simulink model "ICE_Tractor_KRAKER_etrailer_v2_3"  (R2023a)
settings: Solver=VariableStepAuto  StartTime=0.0  StopTime=tmax  FixedStep=dt  RelTol=1e-3  EnableMultiTasking=on
PreLoadFcn:
  | init_vehicle
  | init_SIMULATION_runfile
StartFcn:
  | tic
StopFcn:
  | toc
  | sim_stop_function
  | ICE_Etrailer_Simscape_MBM_plotting
values from neighbouring files (symbols this model uses):
  Arms = [100 200 300 400 500 600]    [init_BURGERS.m]    (also in init_KRAKER.m)
  brake_input = [0   tmax ... (first row only)    [init_vehicle.m]    (also in run_Circle.m = [0  tmax; run_Coastdown.m = [0  2  tmax; run_DoubleLaneChangeDriver.m = [0   2  tmax; run_MaxAcc.m = [0  2  tmax)
  chassis_length = 13.82    [init_BURGERS.m]    (also in init_KRAKER.m = 10.36)
  Diesel_density = 850    [init_BURGERS.m]    (also in init_KRAKER.m)
  Eff = [336.0 370.2 399.2 423.6 444.0 461.0 475.2 487.2 496.2 502.6 506.2 506.9 504.2 500.0 492.4 482.3 469.2 ; 271.0 278.2 285.5 292.8 300.0 307.0 313.7 320.0 325.9 331.5 336.7 341.5 345.9 350.0 353.7 357.0 360.0 ; 223.2 222.7 222.2 221.9 222.0 222.7 224.2 226.7 230.0 234.2 239.3 245.3 252.2 260.0 268.7 278.2 288.7 ; 227.6 221.7 216.8 212.9 210.0 208.1 207.2 207.3 208.5 210.7 214.0 218.3 223.6 230.0 237 ...(+640 chars)    [init_BURGERS.m]    (also in init_KRAKER.m)
  energyCapacity = 116.89    [init_BURGERS.m]    (also in init_KRAKER.m)
  etrailer_ON = 1    [init_SIMULATION_runfile.m]
  front_overhang = 1.620    (= 1.62)    [init_BURGERS.m]    (also in init_KRAKER.m = 1.305)
  G_diff = 1    [init_BURGERS.m]    (also in init_KRAKER.m = 6)
  initialSOC = 0.95    [init_BURGERS.m]    (also in init_KRAKER.m = 0.65)
  InputSwitch = 2    [init_SIMULATION_runfile.m]
  inverter_thermal_res = 0.017    [init_BURGERS.m]    (also in init_KRAKER.m)
  L_0f = 3.8    [init_vehicle.m]
  LD = 1    [init_vehicle.m]
  mass = mass_trailer    (= 11000)    [init_BURGERS.m]    (also in init_KRAKER.m = 7350; run_Statics_MF_MAT.m = (Fz_front_axle1+Fz_rear_axle1+       Fz_trailer1_axle1+Fz_tr; run_Statics_MF_TNO.m = (Fz_front_axle1+Fz_rear_axle1+       Fz_trailer1_axle1+Fz_tr)
  massload = 23000    [init_SIMULATION_runfile.m]
  MaxTrqOut = 525    [init_BURGERS.m]    (also in init_KRAKER.m = 950)
  outside_temp = 25    [init_BURGERS.m]    (also in init_KRAKER.m)
  pose_t0 = [0 0 0 0]    [init_vehicle.m]    (also in run_Circle.m; run_Coastdown.m; run_DoubleLaneChangeDriver.m; run_MaxAcc.m)
  Power_dissipation = [261 384 513 642; 552 783 1020 1260; 894 1233 1584 1956; 1300 1750 2200 2740; 1740 2300 2900 3550; 2250 2900 3650 4500]    [init_BURGERS.m]    (also in init_KRAKER.m)
  RPM = [400 500 600 700 800 900 1000 1100 1200 1300 1400 1500 1600 1700 1800 1900 2000]    [init_BURGERS.m]    (also in init_KRAKER.m)
  sp_t = 0.01    [init_vehicle.m]
  Std_Regen_Trq = 300    [init_BURGERS.m]    (also in init_KRAKER.m)
  steer_input = [0  tmax ... (first row only)    [init_vehicle.m]    (also in run_Circle.m = [0  2   10     13       tmax; run_Coastdown.m = [0 tmax; run_DoubleLaneChangeDriver.m = [0 tmax; run_MaxAcc.m = [0 tmax)
  steer_ratio = 20    [init_vehicle.m]
  steer_sens = 1    [init_vehicle.m]
  throttle_input = [0         tmax ... (first row only)    [init_vehicle.m]    (also in run_Circle.m; run_Coastdown.m = [0        10         10.0001 tmax; run_DoubleLaneChangeDriver.m = [0        tmax; run_MaxAcc.m = [0        tmax)
  tire_param_drive = simscape.multibody.tirread('DRIVE_315_70R22.5_9b_MF62.tir')    [init_vehicle.m]
  tire_param_steer = simscape.multibody.tirread('STEER_315_70R22.5_9b_MF62.tir')    [init_vehicle.m]
  tire_param_trailer = simscape.multibody.tirread('TRAILER_385_65R22.5_9b0_MF62.tir')    [init_vehicle.m]
  tire_width = 0.318    [init_vehicle.m]
  Torq = [0 250 500 750 1000 1250 1500 1750 1850 2000]    [init_BURGERS.m]    (also in init_KRAKER.m)
  trailer_ID = 1    [init_SIMULATION_runfile.m]
  v_0 = 1    [init_vehicle.m]
  Vdc = [200 400 600 800]    [init_BURGERS.m]    (also in init_KRAKER.m)
  Voc = 675    [init_BURGERS.m]    (also in init_KRAKER.m)
  Vx = 0    [init_vehicle.m]    (also in run_Circle.m = Vx_kmh/3.6; run_Coastdown.m = Vx_kmh/3.6; run_DoubleLaneChangeDriver.m = Vx_kmh/3.6; run_MaxAcc.m)
  Vx_input = [0  tmax ... (first row only)    [init_vehicle.m]    (also in run_Circle.m; run_Coastdown.m = [0 tmax; run_DoubleLaneChangeDriver.m = [0 tmax; run_MaxAcc.m = [0 tmax)
  wheelbase = 8.115    [init_BURGERS.m]    (also in init_KRAKER.m = 5.584)
undefined symbols (not defined in the file or in its folder): end_val, final_x, final_y, Floor, steer_path, X, Y, Z
libraries: sm_lib x367, nesl_utility x281, fl_lib x15, sdl_lib x2, robotalgslib x1, simulink_extras x1, batteryecm_lib x1, ee_lib x1, BatteryEstimators x1, CommercialVehicleLibrary2G x1
(part 10 of 14)

== system ICE_Tractor_KRAKER_etrailer_v2_3/Tractor_semitrailer /KRAKER e-trailer/Trailer axle 1/Wheel FR ==
  Bus Creator : BusCreator  Inputs=6
  Bus Creator2 : BusCreator  Inputs=3
  Demux : Demux  Outputs=3
  Demux1 : Demux  Outputs=3
  Geometry Transform : sm_lib/Frames and Transforms/Rigid Transform  TranslationMethod=None  TranslationStandardOffset=0  TranslationStandardOffsetUnits=m  TranslationStandardAxis=+Y  TranslationCartesianOffset=[0 0 0]  TranslationCartesianOffsetUnits=m  TranslationROffset=0  TranslationROffsetUnits=m  TranslationZOffset=0  TranslationZOffsetUnits=m  TranslationThetaOffset=0  TranslationThetaOffsetUnits=deg  RotationMethod=StandardAxis  RotationAngleUnits=deg  RotationStandardAxis=+Z  RotationAngle=sideL*90  RotationArbitraryAxis=[0 0 1]  FollAlignAxisA=+X  BaseAlignAxisA=+Y  FollAlignAxisB=+Y  BaseAlignAxisB=+Z  RotationSequenceAxes=FollowerAxes  RotationSequence=XYX  RotationSequenceAngles=[0 0 0]  RotationSequenceAnglesUnits=deg  RotationMatrix=[1 0 0; 0 1 0; 0 0 1]  Quaternion=[1 0 0 0]
  Inertia : sm_lib/Body Elements/Inertia  InertiaType=Custom  Mass=wheelbody_mass  MassUnits=kg  CenterOfMass=[0 0 0]  CenterOfMassUnits=m  MomentsOfInertia=[Imat(1,1) Imat(2,2) Imat(3,3)]  MomentsOfInertiaUnits=kg*m^2  ProductsOfInertia=[0 0 0]  ProductsOfInertiaUnits=kg*m^2  GraphicType=None  MarkerShape=Inertia  MarkerSize=20  GraphicVisPropType=SimpleVisualProperties  GraphicDiffuseColor=[0.5 0.5 0.5]  GraphicSpecularColor=[0.5 0.5 0.5 1.0]  GraphicAmbientColor=[0.15 0.15 0.15 1.0]  GraphicEmissiveColor=[0.0 0.0 0.0 1.0]  GraphicShininess=75  GraphicOpacity=1.0
  MF Tire FL : sm_lib/Forces and Torques/Magic Formula Tire Force and Torque  TireSide=Right  TireParameters=tire_param  SlipMode=Combined  NumericParameters=[0.1 0.1 0.1 0.1 5.0 1e-4 1e-4 1e-7 1e-7 1e-4 1e-4 0.1 1e-4 1e-4 1e-4 1e-4 1e-4 1e-4 1e-4 1e-4 1e-4]  ScalingCoefficientLMUXMode=FromTireParameters  ScalingCoefficientLMUYMode=FromTireParameters  TireWrenchFrame=ContactFrame  SenseTireForce=on  SenseTireTorque=on  SensePneumaticTrail=off  SenseLongitudinalSlip=off  SenseSaturatedLongitudinalSlip=off  SenseSlipAngle=off  SenseSaturatedSlipAngle=off  SenseTurnSlip=off  SenseRelativeLongitudinalVelocity=off  SenseRelativeLateralVelocity=off  SenseLongitudinalSlipVelocity=off  SenseLateralSlipVelocity=off  SenseYawVelocity=off  SenseCamberAngle=off  SenseSaturatedCamberAngle=off  SenseCamberVelocity=off  SenseSpinVelocity=off  SenseFreeRadius=off  SenseLoadedRadius=off  SenseEffectiveRollingRadius=off  SenseLongitudinalFrictionCoefficient=off  SenseLateralFrictionCoefficient=off  SenseContactBaseRotation=off  SenseContactBaseTranslation=off  SenseContactFollowerRotation=off  SenseContactFollowerTranslation=off
  PS-Simulink Converter : nesl_utility/PS-Simulink Converter  PhysicalDomain=network_engine_domain  SubClassName=ps_output  LeftPortType=input  RightPortType=output  PseudoPeriodic=off  Frequencies=[]  VectorFormat=inherit  Unit=inherit  AffineConversion=off
  PS-Simulink Converter1 : nesl_utility/PS-Simulink Converter  PhysicalDomain=network_engine_domain  SubClassName=ps_output  LeftPortType=input  RightPortType=output  PseudoPeriodic=off  Frequencies=[]  VectorFormat=inherit  Unit=inherit  AffineConversion=off
  PS-Simulink Converter{2..11} (10 alike) : nesl_utility/PS-Simulink Converter  PhysicalDomain=network_engine_domain  SubClassName=ps_output  LeftPortType=input  RightPortType=output  PseudoPeriodic=off  Frequencies=[]  VectorFormat=1-D array  Unit=1  AffineConversion=off
  Reshape : Reshape
  Rigid Transform : sm_lib/Frames and Transforms/Rigid Transform  TranslationMethod=StandardAxis  TranslationStandardOffset=tire_width/2  TranslationStandardOffsetUnits=m  TranslationStandardAxis=-Z  TranslationCartesianOffset=[0 0 0]  TranslationCartesianOffsetUnits=m  TranslationROffset=0  TranslationROffsetUnits=m  TranslationZOffset=0  TranslationZOffsetUnits=m  TranslationThetaOffset=0  TranslationThetaOffsetUnits=deg  RotationMethod=None  RotationAngleUnits=deg  RotationStandardAxis=+Z  RotationAngle=0.0  RotationArbitraryAxis=[0 0 1]  FollAlignAxisA=+X  BaseAlignAxisA=+Y  FollAlignAxisB=+Y  BaseAlignAxisB=+Z  RotationSequenceAxes=FollowerAxes  RotationSequence=XYX  RotationSequenceAngles=[0 0 0]  RotationSequenceAnglesUnits=deg  RotationMatrix=[1 0 0; 0 1 0; 0 0 1]  Quaternion=[1 0 0 0]
  Rim+Tire : sm_lib/Body Elements/File Solid  ExtGeomFileName=wheel.STP  UnitType=Custom  ExtGeomFileUnits=mm  StepReaderType=HEX  ExportConvexHullGeometry=off  InertiaType=Custom  Mass=0  MassUnits=kg  CenterOfMass=[0 0 0]  CenterOfMassUnits=m  MomentsOfInertia=[0 0 0]  MomentsOfInertiaUnits=kg*m^2  ProductsOfInertia=[0 0 0]  ProductsOfInertiaUnits=kg*m^2  BasedOnType=Density  Density=1000  DensityUnits=kg/(m^3)  DoExposeReferenceFrame=on  SerializedFrames=<Frames/>  GraphicType=FromGeometry  MarkerShape=Sphere  MarkerSize=10  GraphicVisPropType=SimpleVisualProperties  GraphicDiffuseColor=[0.8 0.8 0.8]  GraphicSpecularColor=[0.5 0.5 0.5 1.0]  GraphicAmbientColor=[0.15 0.15 0.15 1.0]  GraphicEmissiveColor=[0.0 0.0 0.0 1.0]  GraphicShininess=75  GraphicOpacity=1.0
  Rotation Axis Transform : sm_lib/Frames and Transforms/Rigid Transform  TranslationMethod=None  TranslationStandardOffset=0  TranslationStandardOffsetUnits=m  TranslationStandardAxis=+Z  TranslationCartesianOffset=[0 0 0]  TranslationCartesianOffsetUnits=m  TranslationROffset=0  TranslationROffsetUnits=m  TranslationZOffset=0  TranslationZOffsetUnits=m  TranslationThetaOffset=0  TranslationThetaOffsetUnits=deg  RotationMethod=AlignedAxes  RotationAngleUnits=deg  RotationStandardAxis=-X  RotationAngle=0  RotationArbitraryAxis=[0 0 1]  FollAlignAxisA=+X  BaseAlignAxisA=+X  FollAlignAxisB=+Z  BaseAlignAxisB=+Y  RotationSequenceAxes=FollowerAxes  RotationSequence=XYX  RotationSequenceAngles=[0 0 0]  RotationSequenceAnglesUnits=deg  RotationMatrix=[1 0 0; 0 1 0; 0 0 1]  Quaternion=[1 0 0 0]
  Terminator{,1..6} (7 alike) : Terminator
  Transform Sensor-LocalBodyCS : sm_lib/Frames and Transforms/Transform Sensor  MeasurementFrame=NonRotatingFollower  RotationSequence=XYX  SenseAngle=off  SenseAxis=off  SenseQ=off  SenseR=off  SenseRotationSequence=off  SenseOmegaX=on  SenseOmegaY=on  SenseOmegaZ=on  SenseQDot=off  SenseRDot=off  SenseRotationSequenceDot=off  SenseAlphaX=off  SenseAlphaY=off  SenseAlphaZ=off  SenseQDDot=off  SenseRDDot=off  SenseX=off  SenseY=off  SenseZ=off  SenseRad=off  SenseAzim=off  SenseDist=off  SenseInc=off  SenseXDot=on  SenseYDot=on  SenseZDot=on  SenseRadDot=off  SenseAzimDot=off  SenseDistDot=off  SenseIncDot=off  SenseXDDot=off  SenseYDDot=off  SenseZDDot=off  SenseRadDDot=off  SenseAzimDDot=off  SenseDistDDot=off  SenseIncDDot=off
  Transform Sensor-WorldCS : sm_lib/Frames and Transforms/Transform Sensor  MeasurementFrame=World  RotationSequence=XYX  SenseAngle=off  SenseAxis=off  SenseQ=off  SenseR=on  SenseRotationSequence=off  SenseOmegaX=off  SenseOmegaY=off  SenseOmegaZ=off  SenseQDot=off  SenseRDot=off  SenseRotationSequenceDot=off  SenseAlphaX=off  SenseAlphaY=off  SenseAlphaZ=off  SenseQDDot=off  SenseRDDot=off  SenseX=on  SenseY=on  SenseZ=on  SenseRad=off  SenseAzim=off  SenseDist=off  SenseInc=off  SenseXDot=off  SenseYDot=off  SenseZDot=off  SenseRadDot=off  SenseAzimDot=off  SenseDistDot=off  SenseIncDot=off  SenseXDDot=off  SenseYDDot=off  SenseZDDot=off  SenseRadDDot=off  SenseAzimDDot=off  SenseDistDDot=off  SenseIncDDot=off
  World Frame : sm_lib/Frames and Transforms/World Frame
  "Wheel " : PMIOPort  Side=Left
  Ground : PMIOPort  Port=2  Side=Left
  Tire Foces : Outport
  Tire Position : Outport  Port=2
  wires:
  PS-Simulink Converter/1 -> Demux/1
  Demux/2 -> Bus Creator/2  "Lateral: Fy"
  Bus Creator/1 -> Tire Foces/1
  Demux/3 -> Bus Creator/3  "Normal: Fz"
  PS-Simulink Converter1/1 -> Demux1/1
  Demux1/2 -> Bus Creator/5  "Rolling Resistance: My"
  Demux1/3 -> Bus Creator/6  "Aligning: Mz"
  Demux1/1 -> Bus Creator/4  "Overturning: Mx"
  Demux/1 -> Bus Creator/1  "Longitudinal: Fx"
  PS-Simulink Converter6/1 -> Terminator1/1  "wx"
  PS-Simulink Converter10/1 -> Terminator5/1  "vy"
  PS-Simulink Converter8/1 -> Terminator3/1  "wz"
  PS-Simulink Converter2/1 -> Reshape/1
  PS-Simulink Converter9/1 -> Terminator4/1  "vx"
  PS-Simulink Converter5/1 -> Bus Creator2/3  "z"
  Bus Creator2/1 -> Tire Position/1
  PS-Simulink Converter7/1 -> Terminator2/1  "wy"
  Reshape/1 -> Terminator/1  "R"
  PS-Simulink Converter3/1 -> Bus Creator2/1  "x"
  PS-Simulink Converter4/1 -> Bus Creator2/2  "y"
  PS-Simulink Converter11/1 -> Terminator6/1  "vz"
  connections:
  PS-Simulink Converter1/LConn1 -- MF Tire FL/RConn3
  PS-Simulink Converter/LConn1 -- MF Tire FL/RConn2
  Ground/RConn1 -- MF Tire FL/LConn1
  Transform Sensor-LocalBodyCS/RConn1 -- "Wheel "/RConn1 -- Rotation Axis Transform/RConn1 -- MF Tire FL/RConn1 -- Rigid Transform/LConn1
  Rim+Tire/RConn1 -- Geometry Transform/RConn1
  Geometry Transform/LConn1 -- Inertia/RConn1 -- Rotation Axis Transform/LConn1
  Transform Sensor-LocalBodyCS/LConn1 -- World Frame/RConn1 -- Transform Sensor-WorldCS/LConn1
  Transform Sensor-WorldCS/RConn1 -- Rigid Transform/RConn1
  Transform Sensor-WorldCS/RConn4 -- PS-Simulink Converter4/LConn1
  Transform Sensor-LocalBodyCS/RConn7 -- PS-Simulink Converter11/LConn1
  Transform Sensor-LocalBodyCS/RConn5 -- PS-Simulink Converter9/LConn1
  Transform Sensor-WorldCS/RConn2 -- PS-Simulink Converter2/LConn1
  Transform Sensor-WorldCS/RConn5 -- PS-Simulink Converter5/LConn1
  Transform Sensor-LocalBodyCS/RConn2 -- PS-Simulink Converter6/LConn1
  Transform Sensor-WorldCS/RConn3 -- PS-Simulink Converter3/LConn1
  Transform Sensor-LocalBodyCS/RConn3 -- PS-Simulink Converter7/LConn1
  Transform Sensor-LocalBodyCS/RConn4 -- PS-Simulink Converter8/LConn1
  Transform Sensor-LocalBodyCS/RConn6 -- PS-Simulink Converter10/LConn1

== system ICE_Tractor_KRAKER_etrailer_v2_3/Tractor_semitrailer /KRAKER e-trailer/Trailer axle 2/Brake//Wheel_bearing ==
  Mb : Inport
  Rotational joint around y axis : Subsystem
  axle : PMIOPort  Side=Left
  wheel : PMIOPort  Port=2  Side=Right
  DriveShaftL : PMIOPort  Port=3  Side=Left
  omega : Outport  VectorParamsAs1DForOutWhenUnconnected=off
  wires:
  Rotational joint around y axis/1(Rotational speed) -> omega/1
  Mb/1 -> Rotational joint around y axis/1(Mb)
  connections:
  Rotational joint around y axis/LConn1 -- axle/RConn1
  wheel/RConn1 -- Rotational joint around y axis/RConn1
  DriveShaftL/RConn1 -- Rotational joint around y axis/LConn2

== system ICE_Tractor_KRAKER_etrailer_v2_3/Tractor_semitrailer /KRAKER e-trailer/Trailer axle 2/Brake//Wheel_bearing1 ==
  Mb : Inport
  Rotational joint around y axis : Subsystem
  axle : PMIOPort  Side=Left
  wheel : PMIOPort  Port=2  Side=Right
  DriveShaftR : PMIOPort  Port=3  Side=Left
  omega : Outport  VectorParamsAs1DForOutWhenUnconnected=off
  wires:
  Rotational joint around y axis/1(Rotational speed) -> omega/1
  Mb/1 -> Rotational joint around y axis/1(Mb)
  connections:
  Rotational joint around y axis/LConn1 -- axle/RConn1
  wheel/RConn1 -- Rotational joint around y axis/RConn1
  DriveShaftR/RConn1 -- Rotational joint around y axis/LConn2

== system ICE_Tractor_KRAKER_etrailer_v2_3/Tractor_semitrailer /KRAKER e-trailer/Trailer axle 2/Wheel FL ==
  Bus Creator : BusCreator  Inputs=6
  Bus Creator2 : BusCreator  Inputs=3
  Demux : Demux  Outputs=3
  Demux1 : Demux  Outputs=3
  Geometry Transform : sm_lib/Frames and Transforms/Rigid Transform  TranslationMethod=None  TranslationStandardOffset=0  TranslationStandardOffsetUnits=m  TranslationStandardAxis=+Y  TranslationCartesianOffset=[0 0 0]  TranslationCartesianOffsetUnits=m  TranslationROffset=0  TranslationROffsetUnits=m  TranslationZOffset=0  TranslationZOffsetUnits=m  TranslationThetaOffset=0  TranslationThetaOffsetUnits=deg  RotationMethod=StandardAxis  RotationAngleUnits=deg  RotationStandardAxis=+Z  RotationAngle=sideR*90  RotationArbitraryAxis=[0 0 1]  FollAlignAxisA=+X  BaseAlignAxisA=+Y  FollAlignAxisB=+Y  BaseAlignAxisB=+Z  RotationSequenceAxes=FollowerAxes  RotationSequence=XYX  RotationSequenceAngles=[0 0 0]  RotationSequenceAnglesUnits=deg  RotationMatrix=[1 0 0; 0 1 0; 0 0 1]  Quaternion=[1 0 0 0]
  Inertia : sm_lib/Body Elements/Inertia  InertiaType=Custom  Mass=wheelbody_mass  MassUnits=kg  CenterOfMass=[0 0 0]  CenterOfMassUnits=m  MomentsOfInertia=[Imat(1,1) Imat(2,2) Imat(3,3)]  MomentsOfInertiaUnits=kg*m^2  ProductsOfInertia=[0 0 0]  ProductsOfInertiaUnits=kg*m^2  GraphicType=None  MarkerShape=Inertia  MarkerSize=20  GraphicVisPropType=SimpleVisualProperties  GraphicDiffuseColor=[0.5 0.5 0.5]  GraphicSpecularColor=[0.5 0.5 0.5 1.0]  GraphicAmbientColor=[0.15 0.15 0.15 1.0]  GraphicEmissiveColor=[0.0 0.0 0.0 1.0]  GraphicShininess=75  GraphicOpacity=1.0
  MF Tire FL : sm_lib/Forces and Torques/Magic Formula Tire Force and Torque  TireSide=Left  TireParameters=tire_param  SlipMode=Combined  NumericParameters=[0.1 0.1 0.1 0.1 5.0 1e-4 1e-4 1e-7 1e-7 1e-4 1e-4 0.1 1e-4 1e-4 1e-4 1e-4 1e-4 1e-4 1e-4 1e-4 1e-4]  ScalingCoefficientLMUXMode=FromTireParameters  ScalingCoefficientLMUYMode=FromTireParameters  TireWrenchFrame=ContactFrame  SenseTireForce=on  SenseTireTorque=on  SensePneumaticTrail=off  SenseLongitudinalSlip=off  SenseSaturatedLongitudinalSlip=off  SenseSlipAngle=off  SenseSaturatedSlipAngle=off  SenseTurnSlip=off  SenseRelativeLongitudinalVelocity=off  SenseRelativeLateralVelocity=off  SenseLongitudinalSlipVelocity=off  SenseLateralSlipVelocity=off  SenseYawVelocity=off  SenseCamberAngle=off  SenseSaturatedCamberAngle=off  SenseCamberVelocity=off  SenseSpinVelocity=off  SenseFreeRadius=off  SenseLoadedRadius=off  SenseEffectiveRollingRadius=off  SenseLongitudinalFrictionCoefficient=off  SenseLateralFrictionCoefficient=off  SenseContactBaseRotation=off  SenseContactBaseTranslation=off  SenseContactFollowerRotation=off  SenseContactFollowerTranslation=off
  PS-Simulink Converter : nesl_utility/PS-Simulink Converter  PhysicalDomain=network_engine_domain  SubClassName=ps_output  LeftPortType=input  RightPortType=output  PseudoPeriodic=off  Frequencies=[]  VectorFormat=inherit  Unit=inherit  AffineConversion=off
  PS-Simulink Converter1 : nesl_utility/PS-Simulink Converter  PhysicalDomain=network_engine_domain  SubClassName=ps_output  LeftPortType=input  RightPortType=output  PseudoPeriodic=off  Frequencies=[]  VectorFormat=inherit  Unit=inherit  AffineConversion=off
  PS-Simulink Converter{2..11} (10 alike) : nesl_utility/PS-Simulink Converter  PhysicalDomain=network_engine_domain  SubClassName=ps_output  LeftPortType=input  RightPortType=output  PseudoPeriodic=off  Frequencies=[]  VectorFormat=1-D array  Unit=1  AffineConversion=off
  Reshape : Reshape
  Rigid Transform : sm_lib/Frames and Transforms/Rigid Transform  TranslationMethod=StandardAxis  TranslationStandardOffset=tire_width/2  TranslationStandardOffsetUnits=m  TranslationStandardAxis=+Z  TranslationCartesianOffset=[0 0 0]  TranslationCartesianOffsetUnits=m  TranslationROffset=0  TranslationROffsetUnits=m  TranslationZOffset=0  TranslationZOffsetUnits=m  TranslationThetaOffset=0  TranslationThetaOffsetUnits=deg  RotationMethod=None  RotationAngleUnits=deg  RotationStandardAxis=+Z  RotationAngle=0.0  RotationArbitraryAxis=[0 0 1]  FollAlignAxisA=+X  BaseAlignAxisA=+Y  FollAlignAxisB=+Y  BaseAlignAxisB=+Z  RotationSequenceAxes=FollowerAxes  RotationSequence=XYX  RotationSequenceAngles=[0 0 0]  RotationSequenceAnglesUnits=deg  RotationMatrix=[1 0 0; 0 1 0; 0 0 1]  Quaternion=[1 0 0 0]
  Rim+Tire : sm_lib/Body Elements/File Solid  ExtGeomFileName=wheel.STP  UnitType=Custom  ExtGeomFileUnits=mm  StepReaderType=HEX  ExportConvexHullGeometry=off  InertiaType=Custom  Mass=0  MassUnits=kg  CenterOfMass=[0 0 0]  CenterOfMassUnits=m  MomentsOfInertia=[0 0 0]  MomentsOfInertiaUnits=kg*m^2  ProductsOfInertia=[0 0 0]  ProductsOfInertiaUnits=kg*m^2  BasedOnType=Density  Density=1000  DensityUnits=kg/(m^3)  DoExposeReferenceFrame=on  SerializedFrames=<Frames/>  GraphicType=FromGeometry  MarkerShape=Sphere  MarkerSize=10  GraphicVisPropType=SimpleVisualProperties  GraphicDiffuseColor=[0.8 0.8 0.8]  GraphicSpecularColor=[0.5 0.5 0.5 1.0]  GraphicAmbientColor=[0.15 0.15 0.15 1.0]  GraphicEmissiveColor=[0.0 0.0 0.0 1.0]  GraphicShininess=75  GraphicOpacity=1.0
  Rotation Axis Transform : sm_lib/Frames and Transforms/Rigid Transform  TranslationMethod=None  TranslationStandardOffset=0  TranslationStandardOffsetUnits=m  TranslationStandardAxis=+Z  TranslationCartesianOffset=[0 0 0]  TranslationCartesianOffsetUnits=m  TranslationROffset=0  TranslationROffsetUnits=m  TranslationZOffset=0  TranslationZOffsetUnits=m  TranslationThetaOffset=0  TranslationThetaOffsetUnits=deg  RotationMethod=AlignedAxes  RotationAngleUnits=deg  RotationStandardAxis=-X  RotationAngle=0  RotationArbitraryAxis=[0 0 1]  FollAlignAxisA=+X  BaseAlignAxisA=+X  FollAlignAxisB=+Z  BaseAlignAxisB=+Y  RotationSequenceAxes=FollowerAxes  RotationSequence=XYX  RotationSequenceAngles=[0 0 0]  RotationSequenceAnglesUnits=deg  RotationMatrix=[1 0 0; 0 1 0; 0 0 1]  Quaternion=[1 0 0 0]
  Terminator{,1..6} (7 alike) : Terminator
  Transform Sensor-LocalBodyCS : sm_lib/Frames and Transforms/Transform Sensor  MeasurementFrame=NonRotatingFollower  RotationSequence=XYX  SenseAngle=off  SenseAxis=off  SenseQ=off  SenseR=off  SenseRotationSequence=off  SenseOmegaX=on  SenseOmegaY=on  SenseOmegaZ=on  SenseQDot=off  SenseRDot=off  SenseRotationSequenceDot=off  SenseAlphaX=off  SenseAlphaY=off  SenseAlphaZ=off  SenseQDDot=off  SenseRDDot=off  SenseX=off  SenseY=off  SenseZ=off  SenseRad=off  SenseAzim=off  SenseDist=off  SenseInc=off  SenseXDot=on  SenseYDot=on  SenseZDot=on  SenseRadDot=off  SenseAzimDot=off  SenseDistDot=off  SenseIncDot=off  SenseXDDot=off  SenseYDDot=off  SenseZDDot=off  SenseRadDDot=off  SenseAzimDDot=off  SenseDistDDot=off  SenseIncDDot=off
  Transform Sensor-WorldCS : sm_lib/Frames and Transforms/Transform Sensor  MeasurementFrame=World  RotationSequence=XYX  SenseAngle=off  SenseAxis=off  SenseQ=off  SenseR=on  SenseRotationSequence=off  SenseOmegaX=off  SenseOmegaY=off  SenseOmegaZ=off  SenseQDot=off  SenseRDot=off  SenseRotationSequenceDot=off  SenseAlphaX=off  SenseAlphaY=off  SenseAlphaZ=off  SenseQDDot=off  SenseRDDot=off  SenseX=on  SenseY=on  SenseZ=on  SenseRad=off  SenseAzim=off  SenseDist=off  SenseInc=off  SenseXDot=off  SenseYDot=off  SenseZDot=off  SenseRadDot=off  SenseAzimDot=off  SenseDistDot=off  SenseIncDot=off  SenseXDDot=off  SenseYDDot=off  SenseZDDot=off  SenseRadDDot=off  SenseAzimDDot=off  SenseDistDDot=off  SenseIncDDot=off
  World Frame : sm_lib/Frames and Transforms/World Frame
  "Wheel " : PMIOPort  Side=Left
  Ground : PMIOPort  Port=2  Side=Left
  Tire Foces : Outport
  Tire Position : Outport  Port=2
  wires:
  PS-Simulink Converter/1 -> Demux/1
  Demux/2 -> Bus Creator/2  "Lateral: Fy"
  Bus Creator/1 -> Tire Foces/1
  Demux/3 -> Bus Creator/3  "Normal: Fz"
  PS-Simulink Converter1/1 -> Demux1/1
  Demux1/2 -> Bus Creator/5  "Rolling Resistance: My"
  Demux1/3 -> Bus Creator/6  "Aligning: Mz"
  Demux1/1 -> Bus Creator/4  "Overturning: Mx"
  Demux/1 -> Bus Creator/1  "Longitudinal: Fx"
  PS-Simulink Converter6/1 -> Terminator1/1  "wx"
  PS-Simulink Converter10/1 -> Terminator5/1  "vy"
  PS-Simulink Converter8/1 -> Terminator3/1  "wz"
  PS-Simulink Converter2/1 -> Reshape/1
  PS-Simulink Converter9/1 -> Terminator4/1  "vx"
  PS-Simulink Converter5/1 -> Bus Creator2/3  "z"
  Bus Creator2/1 -> Tire Position/1
  PS-Simulink Converter7/1 -> Terminator2/1  "wy"
  Reshape/1 -> Terminator/1  "R"
  PS-Simulink Converter3/1 -> Bus Creator2/1  "x"
  PS-Simulink Converter4/1 -> Bus Creator2/2  "y"
  PS-Simulink Converter11/1 -> Terminator6/1  "vz"
  connections:
  PS-Simulink Converter1/LConn1 -- MF Tire FL/RConn3
  PS-Simulink Converter/LConn1 -- MF Tire FL/RConn2
  Ground/RConn1 -- MF Tire FL/LConn1
  Transform Sensor-LocalBodyCS/RConn1 -- Rigid Transform/LConn1 -- MF Tire FL/RConn1 -- Rotation Axis Transform/RConn1 -- "Wheel "/RConn1
  Rim+Tire/RConn1 -- Geometry Transform/RConn1
  Geometry Transform/LConn1 -- Inertia/RConn1 -- Rotation Axis Transform/LConn1
  Transform Sensor-LocalBodyCS/LConn1 -- World Frame/RConn1 -- Transform Sensor-WorldCS/LConn1
  Transform Sensor-WorldCS/RConn1 -- Rigid Transform/RConn1
  Transform Sensor-WorldCS/RConn4 -- PS-Simulink Converter4/LConn1
  Transform Sensor-LocalBodyCS/RConn7 -- PS-Simulink Converter11/LConn1
  Transform Sensor-LocalBodyCS/RConn5 -- PS-Simulink Converter9/LConn1
  Transform Sensor-WorldCS/RConn2 -- PS-Simulink Converter2/LConn1
  Transform Sensor-WorldCS/RConn5 -- PS-Simulink Converter5/LConn1
  Transform Sensor-LocalBodyCS/RConn2 -- PS-Simulink Converter6/LConn1
  Transform Sensor-WorldCS/RConn3 -- PS-Simulink Converter3/LConn1
  Transform Sensor-LocalBodyCS/RConn3 -- PS-Simulink Converter7/LConn1
  Transform Sensor-LocalBodyCS/RConn4 -- PS-Simulink Converter8/LConn1
  Transform Sensor-LocalBodyCS/RConn6 -- PS-Simulink Converter10/LConn1

== system ICE_Tractor_KRAKER_etrailer_v2_3/Tractor_semitrailer /KRAKER e-trailer/Trailer axle 2/Wheel FR ==
  Bus Creator : BusCreator  Inputs=6
  Bus Creator2 : BusCreator  Inputs=3
  Demux : Demux  Outputs=3
  Demux1 : Demux  Outputs=3
  Geometry Transform : sm_lib/Frames and Transforms/Rigid Transform  TranslationMethod=None  TranslationStandardOffset=0  TranslationStandardOffsetUnits=m  TranslationStandardAxis=+Y  TranslationCartesianOffset=[0 0 0]  TranslationCartesianOffsetUnits=m  TranslationROffset=0  TranslationROffsetUnits=m  TranslationZOffset=0  TranslationZOffsetUnits=m  TranslationThetaOffset=0  TranslationThetaOffsetUnits=deg  RotationMethod=StandardAxis  RotationAngleUnits=deg  RotationStandardAxis=+Z  RotationAngle=sideL*90  RotationArbitraryAxis=[0 0 1]  FollAlignAxisA=+X  BaseAlignAxisA=+Y  FollAlignAxisB=+Y  BaseAlignAxisB=+Z  RotationSequenceAxes=FollowerAxes  RotationSequence=XYX  RotationSequenceAngles=[0 0 0]  RotationSequenceAnglesUnits=deg  RotationMatrix=[1 0 0; 0 1 0; 0 0 1]  Quaternion=[1 0 0 0]
  Inertia : sm_lib/Body Elements/Inertia  InertiaType=Custom  Mass=wheelbody_mass  MassUnits=kg  CenterOfMass=[0 0 0]  CenterOfMassUnits=m  MomentsOfInertia=[Imat(1,1) Imat(2,2) Imat(3,3)]  MomentsOfInertiaUnits=kg*m^2  ProductsOfInertia=[0 0 0]  ProductsOfInertiaUnits=kg*m^2  GraphicType=None  MarkerShape=Inertia  MarkerSize=20  GraphicVisPropType=SimpleVisualProperties  GraphicDiffuseColor=[0.5 0.5 0.5]  GraphicSpecularColor=[0.5 0.5 0.5 1.0]  GraphicAmbientColor=[0.15 0.15 0.15 1.0]  GraphicEmissiveColor=[0.0 0.0 0.0 1.0]  GraphicShininess=75  GraphicOpacity=1.0
  MF Tire FL : sm_lib/Forces and Torques/Magic Formula Tire Force and Torque  TireSide=Right  TireParameters=tire_param  SlipMode=Combined  NumericParameters=[0.1 0.1 0.1 0.1 5.0 1e-4 1e-4 1e-7 1e-7 1e-4 1e-4 0.1 1e-4 1e-4 1e-4 1e-4 1e-4 1e-4 1e-4 1e-4 1e-4]  ScalingCoefficientLMUXMode=FromTireParameters  ScalingCoefficientLMUYMode=FromTireParameters  TireWrenchFrame=ContactFrame  SenseTireForce=on  SenseTireTorque=on  SensePneumaticTrail=off  SenseLongitudinalSlip=off  SenseSaturatedLongitudinalSlip=off  SenseSlipAngle=off  SenseSaturatedSlipAngle=off  SenseTurnSlip=off  SenseRelativeLongitudinalVelocity=off  SenseRelativeLateralVelocity=off  SenseLongitudinalSlipVelocity=off  SenseLateralSlipVelocity=off  SenseYawVelocity=off  SenseCamberAngle=off  SenseSaturatedCamberAngle=off  SenseCamberVelocity=off  SenseSpinVelocity=off  SenseFreeRadius=off  SenseLoadedRadius=off  SenseEffectiveRollingRadius=off  SenseLongitudinalFrictionCoefficient=off  SenseLateralFrictionCoefficient=off  SenseContactBaseRotation=off  SenseContactBaseTranslation=off  SenseContactFollowerRotation=off  SenseContactFollowerTranslation=off
  PS-Simulink Converter : nesl_utility/PS-Simulink Converter  PhysicalDomain=network_engine_domain  SubClassName=ps_output  LeftPortType=input  RightPortType=output  PseudoPeriodic=off  Frequencies=[]  VectorFormat=inherit  Unit=inherit  AffineConversion=off
  PS-Simulink Converter1 : nesl_utility/PS-Simulink Converter  PhysicalDomain=network_engine_domain  SubClassName=ps_output  LeftPortType=input  RightPortType=output  PseudoPeriodic=off  Frequencies=[]  VectorFormat=inherit  Unit=inherit  AffineConversion=off
  PS-Simulink Converter{2..11} (10 alike) : nesl_utility/PS-Simulink Converter  PhysicalDomain=network_engine_domain  SubClassName=ps_output  LeftPortType=input  RightPortType=output  PseudoPeriodic=off  Frequencies=[]  VectorFormat=1-D array  Unit=1  AffineConversion=off
  Reshape : Reshape
  Rigid Transform : sm_lib/Frames and Transforms/Rigid Transform  TranslationMethod=StandardAxis  TranslationStandardOffset=tire_width/2  TranslationStandardOffsetUnits=m  TranslationStandardAxis=-Z  TranslationCartesianOffset=[0 0 0]  TranslationCartesianOffsetUnits=m  TranslationROffset=0  TranslationROffsetUnits=m  TranslationZOffset=0  TranslationZOffsetUnits=m  TranslationThetaOffset=0  TranslationThetaOffsetUnits=deg  RotationMethod=None  RotationAngleUnits=deg  RotationStandardAxis=+Z  RotationAngle=0.0  RotationArbitraryAxis=[0 0 1]  FollAlignAxisA=+X  BaseAlignAxisA=+Y  FollAlignAxisB=+Y  BaseAlignAxisB=+Z  RotationSequenceAxes=FollowerAxes  RotationSequence=XYX  RotationSequenceAngles=[0 0 0]  RotationSequenceAnglesUnits=deg  RotationMatrix=[1 0 0; 0 1 0; 0 0 1]  Quaternion=[1 0 0 0]
  Rim+Tire : sm_lib/Body Elements/File Solid  ExtGeomFileName=wheel.STP  UnitType=Custom  ExtGeomFileUnits=mm  StepReaderType=HEX  ExportConvexHullGeometry=off  InertiaType=Custom  Mass=0  MassUnits=kg  CenterOfMass=[0 0 0]  CenterOfMassUnits=m  MomentsOfInertia=[0 0 0]  MomentsOfInertiaUnits=kg*m^2  ProductsOfInertia=[0 0 0]  ProductsOfInertiaUnits=kg*m^2  BasedOnType=Density  Density=1000  DensityUnits=kg/(m^3)  DoExposeReferenceFrame=on  SerializedFrames=<Frames/>  GraphicType=FromGeometry  MarkerShape=Sphere  MarkerSize=10  GraphicVisPropType=SimpleVisualProperties  GraphicDiffuseColor=[0.8 0.8 0.8]  GraphicSpecularColor=[0.5 0.5 0.5 1.0]  GraphicAmbientColor=[0.15 0.15 0.15 1.0]  GraphicEmissiveColor=[0.0 0.0 0.0 1.0]  GraphicShininess=75  GraphicOpacity=1.0
  Rotation Axis Transform : sm_lib/Frames and Transforms/Rigid Transform  TranslationMethod=None  TranslationStandardOffset=0  TranslationStandardOffsetUnits=m  TranslationStandardAxis=+Z  TranslationCartesianOffset=[0 0 0]  TranslationCartesianOffsetUnits=m  TranslationROffset=0  TranslationROffsetUnits=m  TranslationZOffset=0  TranslationZOffsetUnits=m  TranslationThetaOffset=0  TranslationThetaOffsetUnits=deg  RotationMethod=AlignedAxes  RotationAngleUnits=deg  RotationStandardAxis=-X  RotationAngle=0  RotationArbitraryAxis=[0 0 1]  FollAlignAxisA=+X  BaseAlignAxisA=+X  FollAlignAxisB=+Z  BaseAlignAxisB=+Y  RotationSequenceAxes=FollowerAxes  RotationSequence=XYX  RotationSequenceAngles=[0 0 0]  RotationSequenceAnglesUnits=deg  RotationMatrix=[1 0 0; 0 1 0; 0 0 1]  Quaternion=[1 0 0 0]
  Terminator{,1..6} (7 alike) : Terminator
  Transform Sensor-LocalBodyCS : sm_lib/Frames and Transforms/Transform Sensor  MeasurementFrame=NonRotatingFollower  RotationSequence=XYX  SenseAngle=off  SenseAxis=off  SenseQ=off  SenseR=off  SenseRotationSequence=off  SenseOmegaX=on  SenseOmegaY=on  SenseOmegaZ=on  SenseQDot=off  SenseRDot=off  SenseRotationSequenceDot=off  SenseAlphaX=off  SenseAlphaY=off  SenseAlphaZ=off  SenseQDDot=off  SenseRDDot=off  SenseX=off  SenseY=off  SenseZ=off  SenseRad=off  SenseAzim=off  SenseDist=off  SenseInc=off  SenseXDot=on  SenseYDot=on  SenseZDot=on  SenseRadDot=off  SenseAzimDot=off  SenseDistDot=off  SenseIncDot=off  SenseXDDot=off  SenseYDDot=off  SenseZDDot=off  SenseRadDDot=off  SenseAzimDDot=off  SenseDistDDot=off  SenseIncDDot=off
  Transform Sensor-WorldCS : sm_lib/Frames and Transforms/Transform Sensor  MeasurementFrame=World  RotationSequence=XYX  SenseAngle=off  SenseAxis=off  SenseQ=off  SenseR=on  SenseRotationSequence=off  SenseOmegaX=off  SenseOmegaY=off  SenseOmegaZ=off  SenseQDot=off  SenseRDot=off  SenseRotationSequenceDot=off  SenseAlphaX=off  SenseAlphaY=off  SenseAlphaZ=off  SenseQDDot=off  SenseRDDot=off  SenseX=on  SenseY=on  SenseZ=on  SenseRad=off  SenseAzim=off  SenseDist=off  SenseInc=off  SenseXDot=off  SenseYDot=off  SenseZDot=off  SenseRadDot=off  SenseAzimDot=off  SenseDistDot=off  SenseIncDot=off  SenseXDDot=off  SenseYDDot=off  SenseZDDot=off  SenseRadDDot=off  SenseAzimDDot=off  SenseDistDDot=off  SenseIncDDot=off
  World Frame : sm_lib/Frames and Transforms/World Frame
  "Wheel " : PMIOPort  Side=Left
  Ground : PMIOPort  Port=2  Side=Left
  Tire Foces : Outport
  Tire Position : Outport  Port=2
  wires:
  PS-Simulink Converter/1 -> Demux/1
  Demux/2 -> Bus Creator/2  "Lateral: Fy"
  Bus Creator/1 -> Tire Foces/1
  Demux/3 -> Bus Creator/3  "Normal: Fz"
  PS-Simulink Converter1/1 -> Demux1/1
  Demux1/2 -> Bus Creator/5  "Rolling Resistance: My"
  Demux1/3 -> Bus Creator/6  "Aligning: Mz"
  Demux1/1 -> Bus Creator/4  "Overturning: Mx"
  Demux/1 -> Bus Creator/1  "Longitudinal: Fx"
  PS-Simulink Converter6/1 -> Terminator1/1  "wx"
  PS-Simulink Converter10/1 -> Terminator5/1  "vy"
  PS-Simulink Converter8/1 -> Terminator3/1  "wz"
  PS-Simulink Converter2/1 -> Reshape/1
  PS-Simulink Converter9/1 -> Terminator4/1  "vx"
  PS-Simulink Converter5/1 -> Bus Creator2/3  "z"
  Bus Creator2/1 -> Tire Position/1
  PS-Simulink Converter7/1 -> Terminator2/1  "wy"
  Reshape/1 -> Terminator/1  "R"
  PS-Simulink Converter3/1 -> Bus Creator2/1  "x"
  PS-Simulink Converter4/1 -> Bus Creator2/2  "y"
  PS-Simulink Converter11/1 -> Terminator6/1  "vz"
  connections:
  PS-Simulink Converter1/LConn1 -- MF Tire FL/RConn3
  PS-Simulink Converter/LConn1 -- MF Tire FL/RConn2
  Ground/RConn1 -- MF Tire FL/LConn1
  Transform Sensor-LocalBodyCS/RConn1 -- "Wheel "/RConn1 -- Rotation Axis Transform/RConn1 -- MF Tire FL/RConn1 -- Rigid Transform/LConn1
  Rim+Tire/RConn1 -- Geometry Transform/RConn1
  Geometry Transform/LConn1 -- Inertia/RConn1 -- Rotation Axis Transform/LConn1
  Transform Sensor-LocalBodyCS/LConn1 -- World Frame/RConn1 -- Transform Sensor-WorldCS/LConn1
  Transform Sensor-WorldCS/RConn1 -- Rigid Transform/RConn1
  Transform Sensor-WorldCS/RConn4 -- PS-Simulink Converter4/LConn1
  Transform Sensor-LocalBodyCS/RConn7 -- PS-Simulink Converter11/LConn1
  Transform Sensor-LocalBodyCS/RConn5 -- PS-Simulink Converter9/LConn1
  Transform Sensor-WorldCS/RConn2 -- PS-Simulink Converter2/LConn1
  Transform Sensor-WorldCS/RConn5 -- PS-Simulink Converter5/LConn1
  Transform Sensor-LocalBodyCS/RConn2 -- PS-Simulink Converter6/LConn1
  Transform Sensor-WorldCS/RConn3 -- PS-Simulink Converter3/LConn1
  Transform Sensor-LocalBodyCS/RConn3 -- PS-Simulink Converter7/LConn1
  Transform Sensor-LocalBodyCS/RConn4 -- PS-Simulink Converter8/LConn1
  Transform Sensor-LocalBodyCS/RConn6 -- PS-Simulink Converter10/LConn1

== system ICE_Tractor_KRAKER_etrailer_v2_3/Tractor_semitrailer /KRAKER e-trailer/Trailer axle 3/Brake//Wheel_bearing ==
  Mdrive : Inport
  Mbrake : Inport  Port=2
  Gain : Gain  Gain=-1
  Look-Up Table : Lookup  InputValues=[-5:0.05:5]  Table=-tanh(2*[-5:0.05:5])
  Product1 : Product  InputSameDT=on  SaturateOnIntegerOverflow=on  OutDataTypeStr=Inherit: Same as first input
  Rotational joint around y axis : Subsystem
  Scope : Scope
  Sum : Sum  Inputs=++|
  axle : PMIOPort  Side=Left
  wheel : PMIOPort  Port=2  Side=Right
  omega : Outport  VectorParamsAs1DForOutWhenUnconnected=off
  wires:
  Mbrake/1 -> Gain/1
  Look-Up Table/1 -> Product1/2
  Product1/1 -> Sum/2
  Mdrive/1 -> Sum/1
  Rotational joint around y axis/1(Rotational speed) -> omega/1, Look-Up Table/1
  Sum/1 -> Rotational joint around y axis/1(Torque), Scope/1
  Gain/1 -> Product1/1
  connections:
  Rotational joint around y axis/LConn1 -- axle/RConn1
  wheel/RConn1 -- Rotational joint around y axis/RConn1

== system ICE_Tractor_KRAKER_etrailer_v2_3/Tractor_semitrailer /KRAKER e-trailer/Trailer axle 3/Brake//Wheel_bearing1 ==
  Mdrive : Inport
  Mbrake : Inport  Port=2
  Gain : Gain  Gain=-1
  Look-Up Table : Lookup  InputValues=[-5:0.05:5]  Table=-tanh(2*[-5:0.05:5])
  Product1 : Product  InputSameDT=on  SaturateOnIntegerOverflow=on  OutDataTypeStr=Inherit: Same as first input
  Rotational joint around y axis : Subsystem
  Sum : Sum  Inputs=++|
  axle : PMIOPort  Side=Left
  wheel : PMIOPort  Port=2  Side=Right
  omega : Outport  VectorParamsAs1DForOutWhenUnconnected=off
  wires:
  Mbrake/1 -> Gain/1
  Look-Up Table/1 -> Product1/2
  Product1/1 -> Sum/2
  Mdrive/1 -> Sum/1
  Rotational joint around y axis/1(Rotational speed) -> omega/1, Look-Up Table/1
  Sum/1 -> Rotational joint around y axis/1(Torque)
  Gain/1 -> Product1/1
  connections:
  Rotational joint around y axis/LConn1 -- axle/RConn1
  wheel/RConn1 -- Rotational joint around y axis/RConn1

== system ICE_Tractor_KRAKER_etrailer_v2_3/Tractor_semitrailer /KRAKER e-trailer/Trailer axle 3/Wheel FL ==
  Bus Creator : BusCreator  Inputs=6
  Bus Creator2 : BusCreator  Inputs=3
  Demux : Demux  Outputs=3
  Demux1 : Demux  Outputs=3
  Geometry Transform : sm_lib/Frames and Transforms/Rigid Transform  TranslationMethod=None  TranslationStandardOffset=0  TranslationStandardOffsetUnits=m  TranslationStandardAxis=+Y  TranslationCartesianOffset=[0 0 0]  TranslationCartesianOffsetUnits=m  TranslationROffset=0  TranslationROffsetUnits=m  TranslationZOffset=0  TranslationZOffsetUnits=m  TranslationThetaOffset=0  TranslationThetaOffsetUnits=deg  RotationMethod=StandardAxis  RotationAngleUnits=deg  RotationStandardAxis=+Z  RotationAngle=sideR*90  RotationArbitraryAxis=[0 0 1]  FollAlignAxisA=+X  BaseAlignAxisA=+Y  FollAlignAxisB=+Y  BaseAlignAxisB=+Z  RotationSequenceAxes=FollowerAxes  RotationSequence=XYX  RotationSequenceAngles=[0 0 0]  RotationSequenceAnglesUnits=deg  RotationMatrix=[1 0 0; 0 1 0; 0 0 1]  Quaternion=[1 0 0 0]
  Inertia : sm_lib/Body Elements/Inertia  InertiaType=Custom  Mass=wheelbody_mass  MassUnits=kg  CenterOfMass=[0 0 0]  CenterOfMassUnits=m  MomentsOfInertia=[Imat(1,1) Imat(2,2) Imat(3,3)]  MomentsOfInertiaUnits=kg*m^2  ProductsOfInertia=[0 0 0]  ProductsOfInertiaUnits=kg*m^2  GraphicType=None  MarkerShape=Inertia  MarkerSize=20  GraphicVisPropType=SimpleVisualProperties  GraphicDiffuseColor=[0.5 0.5 0.5]  GraphicSpecularColor=[0.5 0.5 0.5 1.0]  GraphicAmbientColor=[0.15 0.15 0.15 1.0]  GraphicEmissiveColor=[0.0 0.0 0.0 1.0]  GraphicShininess=75  GraphicOpacity=1.0
  MF Tire FL : sm_lib/Forces and Torques/Magic Formula Tire Force and Torque  TireSide=Left  TireParameters=tire_param  SlipMode=Combined  NumericParameters=[0.1 0.1 0.1 0.1 5.0 1e-4 1e-4 1e-7 1e-7 1e-4 1e-4 0.1 1e-4 1e-4 1e-4 1e-4 1e-4 1e-4 1e-4 1e-4 1e-4]  ScalingCoefficientLMUXMode=FromTireParameters  ScalingCoefficientLMUYMode=FromTireParameters  TireWrenchFrame=ContactFrame  SenseTireForce=on  SenseTireTorque=on  SensePneumaticTrail=off  SenseLongitudinalSlip=off  SenseSaturatedLongitudinalSlip=off  SenseSlipAngle=off  SenseSaturatedSlipAngle=off  SenseTurnSlip=off  SenseRelativeLongitudinalVelocity=off  SenseRelativeLateralVelocity=off  SenseLongitudinalSlipVelocity=off  SenseLateralSlipVelocity=off  SenseYawVelocity=off  SenseCamberAngle=off  SenseSaturatedCamberAngle=off  SenseCamberVelocity=off  SenseSpinVelocity=off  SenseFreeRadius=off  SenseLoadedRadius=off  SenseEffectiveRollingRadius=off  SenseLongitudinalFrictionCoefficient=off  SenseLateralFrictionCoefficient=off  SenseContactBaseRotation=off  SenseContactBaseTranslation=off  SenseContactFollowerRotation=off  SenseContactFollowerTranslation=off
  PS-Simulink Converter : nesl_utility/PS-Simulink Converter  PhysicalDomain=network_engine_domain  SubClassName=ps_output  LeftPortType=input  RightPortType=output  PseudoPeriodic=off  Frequencies=[]  VectorFormat=inherit  Unit=inherit  AffineConversion=off
  PS-Simulink Converter1 : nesl_utility/PS-Simulink Converter  PhysicalDomain=network_engine_domain  SubClassName=ps_output  LeftPortType=input  RightPortType=output  PseudoPeriodic=off  Frequencies=[]  VectorFormat=inherit  Unit=inherit  AffineConversion=off
  PS-Simulink Converter{2..11} (10 alike) : nesl_utility/PS-Simulink Converter  PhysicalDomain=network_engine_domain  SubClassName=ps_output  LeftPortType=input  RightPortType=output  PseudoPeriodic=off  Frequencies=[]  VectorFormat=1-D array  Unit=1  AffineConversion=off
  Reshape : Reshape
  Rigid Transform : sm_lib/Frames and Transforms/Rigid Transform  TranslationMethod=StandardAxis  TranslationStandardOffset=tire_width/2  TranslationStandardOffsetUnits=m  TranslationStandardAxis=+Z  TranslationCartesianOffset=[0 0 0]  TranslationCartesianOffsetUnits=m  TranslationROffset=0  TranslationROffsetUnits=m  TranslationZOffset=0  TranslationZOffsetUnits=m  TranslationThetaOffset=0  TranslationThetaOffsetUnits=deg  RotationMethod=None  RotationAngleUnits=deg  RotationStandardAxis=+Z  RotationAngle=0.0  RotationArbitraryAxis=[0 0 1]  FollAlignAxisA=+X  BaseAlignAxisA=+Y  FollAlignAxisB=+Y  BaseAlignAxisB=+Z  RotationSequenceAxes=FollowerAxes  RotationSequence=XYX  RotationSequenceAngles=[0 0 0]  RotationSequenceAnglesUnits=deg  RotationMatrix=[1 0 0; 0 1 0; 0 0 1]  Quaternion=[1 0 0 0]
  Rim+Tire : sm_lib/Body Elements/File Solid  ExtGeomFileName=wheel.STP  UnitType=Custom  ExtGeomFileUnits=mm  StepReaderType=HEX  ExportConvexHullGeometry=off  InertiaType=Custom  Mass=0  MassUnits=kg  CenterOfMass=[0 0 0]  CenterOfMassUnits=m  MomentsOfInertia=[0 0 0]  MomentsOfInertiaUnits=kg*m^2  ProductsOfInertia=[0 0 0]  ProductsOfInertiaUnits=kg*m^2  BasedOnType=Density  Density=1000  DensityUnits=kg/(m^3)  DoExposeReferenceFrame=on  SerializedFrames=<Frames/>  GraphicType=FromGeometry  MarkerShape=Sphere  MarkerSize=10  GraphicVisPropType=SimpleVisualProperties  GraphicDiffuseColor=[0.8 0.8 0.8]  GraphicSpecularColor=[0.5 0.5 0.5 1.0]  GraphicAmbientColor=[0.15 0.15 0.15 1.0]  GraphicEmissiveColor=[0.0 0.0 0.0 1.0]  GraphicShininess=75  GraphicOpacity=1.0
  Rotation Axis Transform : sm_lib/Frames and Transforms/Rigid Transform  TranslationMethod=None  TranslationStandardOffset=0  TranslationStandardOffsetUnits=m  TranslationStandardAxis=+Z  TranslationCartesianOffset=[0 0 0]  TranslationCartesianOffsetUnits=m  TranslationROffset=0  TranslationROffsetUnits=m  TranslationZOffset=0  TranslationZOffsetUnits=m  TranslationThetaOffset=0  TranslationThetaOffsetUnits=deg  RotationMethod=AlignedAxes  RotationAngleUnits=deg  RotationStandardAxis=-X  RotationAngle=0  RotationArbitraryAxis=[0 0 1]  FollAlignAxisA=+X  BaseAlignAxisA=+X  FollAlignAxisB=+Z  BaseAlignAxisB=+Y  RotationSequenceAxes=FollowerAxes  RotationSequence=XYX  RotationSequenceAngles=[0 0 0]  RotationSequenceAnglesUnits=deg  RotationMatrix=[1 0 0; 0 1 0; 0 0 1]  Quaternion=[1 0 0 0]
  Terminator{,1..6} (7 alike) : Terminator
  Transform Sensor-LocalBodyCS : sm_lib/Frames and Transforms/Transform Sensor  MeasurementFrame=NonRotatingFollower  RotationSequence=XYX  SenseAngle=off  SenseAxis=off  SenseQ=off  SenseR=off  SenseRotationSequence=off  SenseOmegaX=on  SenseOmegaY=on  SenseOmegaZ=on  SenseQDot=off  SenseRDot=off  SenseRotationSequenceDot=off  SenseAlphaX=off  SenseAlphaY=off  SenseAlphaZ=off  SenseQDDot=off  SenseRDDot=off  SenseX=off  SenseY=off  SenseZ=off  SenseRad=off  SenseAzim=off  SenseDist=off  SenseInc=off  SenseXDot=on  SenseYDot=on  SenseZDot=on  SenseRadDot=off  SenseAzimDot=off  SenseDistDot=off  SenseIncDot=off  SenseXDDot=off  SenseYDDot=off  SenseZDDot=off  SenseRadDDot=off  SenseAzimDDot=off  SenseDistDDot=off  SenseIncDDot=off
  Transform Sensor-WorldCS : sm_lib/Frames and Transforms/Transform Sensor  MeasurementFrame=World  RotationSequence=XYX  SenseAngle=off  SenseAxis=off  SenseQ=off  SenseR=on  SenseRotationSequence=off  SenseOmegaX=off  SenseOmegaY=off  SenseOmegaZ=off  SenseQDot=off  SenseRDot=off  SenseRotationSequenceDot=off  SenseAlphaX=off  SenseAlphaY=off  SenseAlphaZ=off  SenseQDDot=off  SenseRDDot=off  SenseX=on  SenseY=on  SenseZ=on  SenseRad=off  SenseAzim=off  SenseDist=off  SenseInc=off  SenseXDot=off  SenseYDot=off  SenseZDot=off  SenseRadDot=off  SenseAzimDot=off  SenseDistDot=off  SenseIncDot=off  SenseXDDot=off  SenseYDDot=off  SenseZDDot=off  SenseRadDDot=off  SenseAzimDDot=off  SenseDistDDot=off  SenseIncDDot=off
  World Frame : sm_lib/Frames and Transforms/World Frame
  "Wheel " : PMIOPort  Side=Left
  Ground : PMIOPort  Port=2  Side=Left
  Tire Foces : Outport
  Tire Position : Outport  Port=2
  wires:
  PS-Simulink Converter/1 -> Demux/1
  Demux/2 -> Bus Creator/2  "Lateral: Fy"
  Bus Creator/1 -> Tire Foces/1
  Demux/3 -> Bus Creator/3  "Normal: Fz"
  PS-Simulink Converter1/1 -> Demux1/1
  Demux1/2 -> Bus Creator/5  "Rolling Resistance: My"
  Demux1/3 -> Bus Creator/6  "Aligning: Mz"
  Demux1/1 -> Bus Creator/4  "Overturning: Mx"
  Demux/1 -> Bus Creator/1  "Longitudinal: Fx"
  PS-Simulink Converter6/1 -> Terminator1/1  "wx"
  PS-Simulink Converter10/1 -> Terminator5/1  "vy"
  PS-Simulink Converter8/1 -> Terminator3/1  "wz"
  PS-Simulink Converter2/1 -> Reshape/1
  PS-Simulink Converter9/1 -> Terminator4/1  "vx"
  PS-Simulink Converter5/1 -> Bus Creator2/3  "z"
  Bus Creator2/1 -> Tire Position/1
  PS-Simulink Converter7/1 -> Terminator2/1  "wy"
  Reshape/1 -> Terminator/1  "R"
  PS-Simulink Converter3/1 -> Bus Creator2/1  "x"
  PS-Simulink Converter4/1 -> Bus Creator2/2  "y"
  PS-Simulink Converter11/1 -> Terminator6/1  "vz"
  connections:
  PS-Simulink Converter1/LConn1 -- MF Tire FL/RConn3
  PS-Simulink Converter/LConn1 -- MF Tire FL/RConn2
  Ground/RConn1 -- MF Tire FL/LConn1
  Transform Sensor-LocalBodyCS/RConn1 -- Rotation Axis Transform/RConn1 -- "Wheel "/RConn1 -- MF Tire FL/RConn1 -- Rigid Transform/LConn1
  Rim+Tire/RConn1 -- Geometry Transform/RConn1
  Geometry Transform/LConn1 -- Inertia/RConn1 -- Rotation Axis Transform/LConn1
  Transform Sensor-LocalBodyCS/LConn1 -- World Frame/RConn1 -- Transform Sensor-WorldCS/LConn1
  Transform Sensor-WorldCS/RConn1 -- Rigid Transform/RConn1
  Transform Sensor-WorldCS/RConn4 -- PS-Simulink Converter4/LConn1
  Transform Sensor-LocalBodyCS/RConn7 -- PS-Simulink Converter11/LConn1
  Transform Sensor-LocalBodyCS/RConn5 -- PS-Simulink Converter9/LConn1
  Transform Sensor-WorldCS/RConn2 -- PS-Simulink Converter2/LConn1
  Transform Sensor-WorldCS/RConn5 -- PS-Simulink Converter5/LConn1
  Transform Sensor-LocalBodyCS/RConn2 -- PS-Simulink Converter6/LConn1
  Transform Sensor-WorldCS/RConn3 -- PS-Simulink Converter3/LConn1
  Transform Sensor-LocalBodyCS/RConn3 -- PS-Simulink Converter7/LConn1
  Transform Sensor-LocalBodyCS/RConn4 -- PS-Simulink Converter8/LConn1
  Transform Sensor-LocalBodyCS/RConn6 -- PS-Simulink Converter10/LConn1
